simulink model "Control - Scenario 3"  (R2019b)
settings: Solver=VariableStepAuto  StartTime=0.0  StopTime=10.0  RelTol=1e-3
libraries: cstblocks x24
settings Model: Creator=Gioele  LastModifiedBy=Gioele

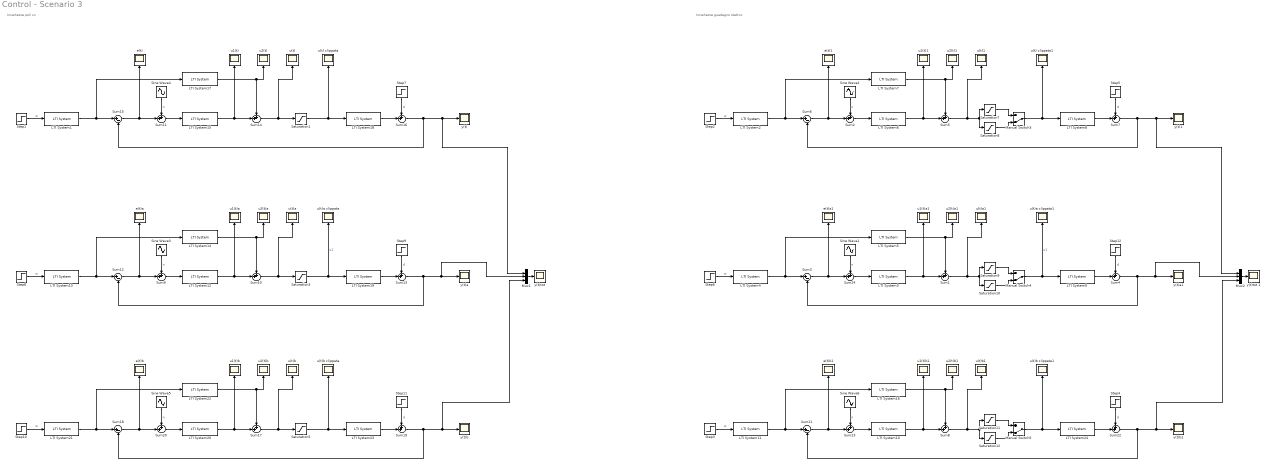
== system Control - Scenario 3 ==
  note: Incertezze guadagno statico
  note: Incertezze poli cc
  LTI System{1..2,4,11,13,21} (6 alike) : cstblocks/LTI System  sys=Rpf_3  IC=[]
  LTI System{3,6,10,12,15,20} (6 alike) : cstblocks/LTI System  sys=R_3  IC=[]
  LTI System{5,7,14,16..17,22} (6 alike) : cstblocks/LTI System  sys=Rff_3  IC=[]
  LTI System18 : cstblocks/LTI System  sys=G  IC=[]
  LTI System19 : cstblocks/LTI System  sys=Ga  IC=[]
  LTI System23 : cstblocks/LTI System  sys=Gb  IC=[]
  LTI System24 : cstblocks/LTI System  sys=Gd  IC=[]
  LTI System8 : cstblocks/LTI System  sys=G  IC=[]
  LTI System9 : cstblocks/LTI System  sys=Gc  IC=[]
  Manual Switch3 : ManualSwitch  CurrentSetting=0
  Manual Switch4 : ManualSwitch  CurrentSetting=0
  Manual Switch5 : ManualSwitch  CurrentSetting=0
  Mux1 : Mux  Inputs=3
  Mux2 : Mux  Inputs=3
  Saturation{1,3,5,7,9,11} (6 alike) : Saturate  UpperLimit=1.9  LowerLimit=-1.9
  Saturation10 : Saturate  UpperLimit=2.1  LowerLimit=-2.1
  Saturation12 : Saturate  UpperLimit=2.1  LowerLimit=-2.1
  Saturation8 : Saturate  UpperLimit=2.1  LowerLimit=-2.1
  Sine Wave{1..6} (6 alike) : Sin  Amplitude=0.005  Frequency=2000  SampleTime=0
  Step{1..3,6,8,10} (6 alike) : Step  Time=0  After=2  SampleTime=0
  Step{4..5,7,9,11..12} (6 alike) : Step  Time=0  After=0.1  SampleTime=0
  Sum{1..2,4..5,7..11,13..14,16..17,19..20,22..24} (18 alike) : Sum  Inputs=++|
  Sum{3,6,12,15,18,21} (6 alike) : Sum  Inputs=|+-
  e(t) : Scope
  e(t)1 : Scope
  e(t)a : Scope
  e(t)a1 : Scope
  e(t)b : Scope
  e(t)b1 : Scope
  u(t) : Scope
  u(t) clippata : Scope
  u(t) clippata1 : Scope
  u(t)1 : Scope
  u(t)a : Scope
  u(t)a clippata : Scope
  u(t)a clippata1 : Scope
  u(t)a1 : Scope
  u(t)b : Scope
  u(t)b clippata : Scope
  u(t)b clippata1 : Scope
  u(t)b1 : Scope
  u1(t) : Scope
  u1(t)1 : Scope
  u1(t)a : Scope
  u1(t)a1 : Scope
  u1(t)b : Scope
  u1(t)b1 : Scope
  u2(t) : Scope
  u2(t)1 : Scope
  u2(t)a : Scope
  u2(t)a1 : Scope
  u2(t)b : Scope
  u2(t)b1 : Scope
  y(t) : Scope
  y(t)1 : Scope
  y(t)a : Scope
  y(t)a1 : Scope
  y(t)b : Scope
  y(t)b1 : Scope
  "y(t)tot " : Scope
  y(t)tot 1 : Scope
  wires:
  Sum12/1 -> e(t)a/1, Sum9/2
  Step9/1 -> Sum13/1  "d"
  Sum9/1 -> LTI System12/1
  LTI System23/1 -> Sum19/2
  Sine Wave5/1 -> Sum20/1  "n"
  LTI System20/1 -> u1(t)b/1, Sum17/2
  Sum11/1 -> LTI System15/1
  LTI System15/1 -> u1(t)/1, Sum14/2
  LTI System18/1 -> Sum16/2
  Step8/1 -> LTI System13/1  "w"
  Sum18/1 -> e(t)b/1, Sum20/2
  LTI System21/1 -> LTI System22/1, Sum18/1
  Step10/1 -> LTI System21/1  "w"
  Sum20/1 -> LTI System20/1
  Sum16/1 -> Sum15/2, Mux1/1, y(t)/1
  Sum19/1 -> Sum18/2, Mux1/3, y(t)b/1
  Step11/1 -> Sum19/1  "d"
  LTI System12/1 -> u1(t)a/1, Sum10/2
  Saturation5/1 -> u(t)b clippata/1, LTI System23/1
  LTI System22/1 -> Sum17/1, u2(t)b/1
  Sine Wave4/1 -> Sum11/1  "n"
  Sum13/1 -> Sum12/2, Mux1/2, y(t)a/1
  LTI System17/1 -> Sum14/1, u2(t)/1
  Mux1/1 -> "y(t)tot "/1
  LTI System14/1 -> Sum10/1, u2(t)a/1
  LTI System19/1 -> Sum13/2
  Saturation3/1 -> u(t)a clippata/1, LTI System19/1  "u1"
  Step1/1 -> LTI System1/1  "w"
  LTI System1/1 -> LTI System17/1, Sum15/1
  Step7/1 -> Sum16/1  "d"
  LTI System13/1 -> LTI System14/1, Sum12/1
  Sum15/1 -> e(t)/1, Sum11/2
  Sine Wave3/1 -> Sum9/1  "n"
  Sum14/1 -> u(t)/1, Saturation1/1
  Saturation1/1 -> u(t) clippata/1, LTI System18/1
  Sum10/1 -> Saturation3/1, u(t)a/1
  Sum17/1 -> u(t)b/1, Saturation5/1
  Sum22/1 -> Sum21/2, Mux2/3, y(t)b1/1
  Manual Switch3/1 -> u(t) clippata1/1, LTI System8/1
  Sum5/1 -> u(t)1/1, Saturation8/1, Saturation7/1
  Saturation12/1 -> Manual Switch5/2
  Saturation11/1 -> Manual Switch5/1
  Saturation9/1 -> Manual Switch4/1
  Sum8/1 -> Saturation12/1, Saturation11/1, u(t)b1/1
  LTI System7/1 -> Sum5/1, u2(t)1/1
  Sine Wave1/1 -> Sum24/1  "n"
  Step5/1 -> Sum7/1  "d"
  Saturation10/1 -> Manual Switch4/2
  Manual Switch5/1 -> u(t)b clippata1/1, LTI System24/1
  LTI System5/1 -> Sum1/1, u2(t)a1/1
  Sum1/1 -> Saturation10/1, Saturation9/1, u(t)a1/1
  LTI System16/1 -> Sum8/1, u2(t)b1/1
  LTI System2/1 -> LTI System7/1, Sum6/1
  Saturation7/1 -> Manual Switch3/1
  Saturation8/1 -> Manual Switch3/2
  Manual Switch4/1 -> u(t)a clippata1/1, LTI System9/1  "u1"
  Mux2/1 -> y(t)tot 1/1
  LTI System9/1 -> Sum4/2
  LTI System3/1 -> u1(t)a1/1, Sum1/2
  LTI System4/1 -> LTI System5/1, Sum3/1
  Sine Wave2/1 -> Sum2/1  "n"
  Sum21/1 -> e(t)b1/1, Sum23/2
  Step6/1 -> LTI System4/1  "w"
  LTI System8/1 -> Sum7/2
  Step2/1 -> LTI System2/1  "w"
  Step12/1 -> Sum4/1  "d"
  LTI System10/1 -> u1(t)b1/1, Sum8/2
  Sum4/1 -> Sum3/2, Mux2/2, y(t)a1/1
  LTI System11/1 -> LTI System16/1, Sum21/1
  Sum6/1 -> e(t)1/1, Sum2/2
  Step4/1 -> Sum22/1  "d"
  LTI System6/1 -> u1(t)1/1, Sum5/2
  Sine Wave6/1 -> Sum23/1  "n"
  Sum7/1 -> Sum6/2, Mux2/1, y(t)1/1
  Sum23/1 -> LTI System10/1
  Sum2/1 -> LTI System6/1
  Sum24/1 -> LTI System3/1
  Sum3/1 -> e(t)a1/1, Sum24/2
  Step3/1 -> LTI System11/1  "w"
  LTI System24/1 -> Sum22/2
